simulink model "motor"  (R2020b)
settings: Solver=ode45  StartTime=0.0  StopTime=33  RelTol=1e-3  EnableMultiTasking=on
PreLoadFcn:
  | MotorParam
InitFcn:
  | MotorParam
values from neighbouring files (symbols this model uses):
  B = (Km*INL)/w    (= 5.6014073536e-07)    [MotorParam.m]
  J = Rotor_inertia    (= 5.33664e-07)    [MotorParam.m]
  Kb = (Speed_constant)/(.10472)    (= 0.0279218545472)    [MotorParam.m]
  Km = Torque_constant*1E-3    (= 0.028)    [MotorParam.m]
  L = Terminal_inductance*1E-3    (= 0.000535)    [MotorParam.m]
  R = Terminal_resistance    (= 8.75)    [MotorParam.m]
libraries: simulink x1
settings Model: Creator=Leo  LastModifiedBy=Jeff
settings DataIOCC: LimitDataPoints=on  SaveFormat=Array  SignalLoggingSaveFormat=ModelDataLogs  ReturnWorkspaceOutputs=off
settings OptimizationCC: ExpressionDepthLimit=2147483647  InitFltsAndDblsToZero=on  LifeSpan=inf
settings DebuggingCC: UnderspecifiedInitializationDetection=Classic  MergeDetectMultiDrivingBlocksExec=none  SolverPrmCheckMsg=warning  FcnCallInpInsideContextMsg=warning  StateNameClashWarn=warning  SFUnexpectedBacktrackingDiag=warning  SFNoUnconditionalDefaultTransitionDiag=warning  SFExecutionAtInitializationDiag=none  ArithmeticOperatorsInVariantConditions=warning
settings HardwareCC: ProdBitPerPointer=32  ProdBitPerSizeT=32  ProdBitPerPtrDiffT=32  ProdLargestAtomicFloat=None  ProdIntDivRoundTo=Undefined  ProdEndianess=Unspecified  ProdWordSize=32  ProdHWDeviceType=32-bit Generic
settings ModelReferenceCC: PropagateSignalLabelsOutOfModel=off
settings SFSimCC: SimUseLocalCustomCode=off  CustomCodeUndefinedFunction=UseInterfaceOnly
settings RTWCC: RTWUseLocalCustomCode=off
settings CodeAppCC: StateflowObjectComments=on
settings GRTTargetCC: TargetLangStandard=C89/C90 (ANSI)  CombineOutputUpdateFcns=off  GRTInterface=on
settings ConfigComp: CovMetricSettings=dw  CovSaveCumulativeToWorkspaceVar=on  CovSaveSingleToWorkspaceVar=on  CovExternalEMLEnable=off  CovSFcnEnable=off

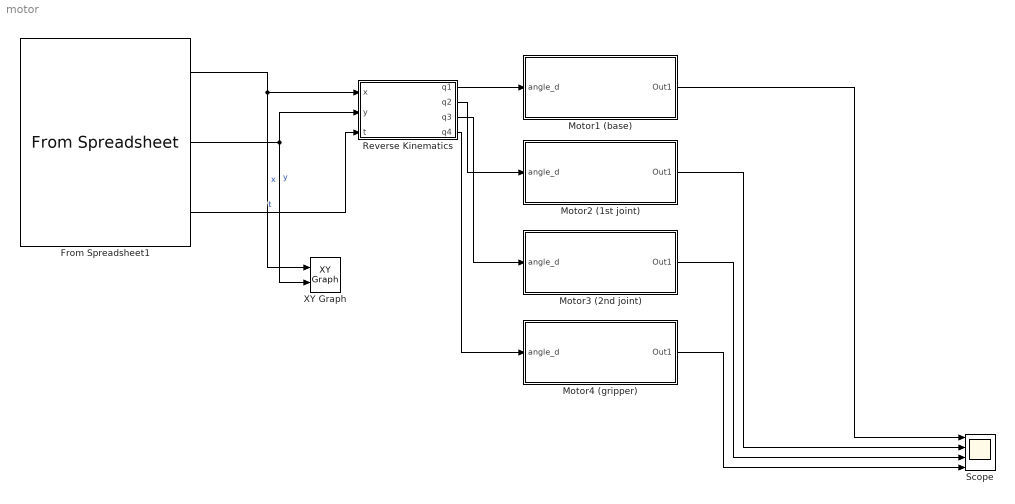
== system motor ==
  From Spreadsheet1 : FromSpreadsheet  FileName=Motor_pos.xlsx
  Motor1 (base) : Subsystem
  Motor2 (1st joint) : Subsystem
  Motor3 (2nd joint) : Subsystem
  Motor4 (gripper) : Subsystem
  Reverse Kinematics : MATLAB Function  TreatAsAtomicUnit=on
  Scope : Scope  NumInputPorts=4
  XY Graph : simulink/Sinks/XY Graph  xmin=-15  xmax=15  ymin=-5  ymax=50  st=0.001
  wires:
  From Spreadsheet1/1 -> XY Graph/1, Reverse Kinematics/1(x)  "x"
  Motor1 (base)/1(Out1) -> Scope/1
  From Spreadsheet1/2 -> XY Graph/2, Reverse Kinematics/2(y)  "y"
  Reverse Kinematics/1(q1) -> Motor1 (base)/1(angle_d)
  Reverse Kinematics/2(q2) -> Motor2 (1st joint)/1(angle_d)
  Reverse Kinematics/3(q3) -> Motor3 (2nd joint)/1(angle_d)
  Motor2 (1st joint)/1(Out1) -> Scope/2
  Motor3 (2nd joint)/1(Out1) -> Scope/3
  Reverse Kinematics/4(q4) -> Motor4 (gripper)/1(angle_d)
  Motor4 (gripper)/1(Out1) -> Scope/4
  From Spreadsheet1/3 -> Reverse Kinematics/3(t)  "t"

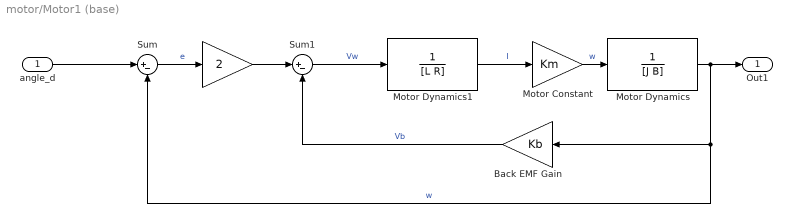
== system motor/Motor1 (base) ==
  angle_d : Inport
  " " : Gain  Gain=2
  Back EMF Gain : Gain  Gain=Kb
  Motor Constant : Gain  Gain=Km
  Motor Dynamics : TransferFcn  Denominator=[J B]
  Motor Dynamics1 : TransferFcn  Denominator=[L R]
  Sum : Sum  Inputs=|+-
  Sum1 : Sum  Inputs=|+-
  Out1 : Outport
  wires:
  angle_d/1 -> Sum/1
  Sum/1 -> " "/1  "e"
  Motor Constant/1 -> Motor Dynamics/1  "w"
  " "/1 -> Sum1/1
  Back EMF Gain/1 -> Sum1/2  "Vb"
  Motor Dynamics1/1 -> Motor Constant/1  "I"
  Sum1/1 -> Motor Dynamics1/1  "Vw"
  Motor Dynamics/1 -> Back EMF Gain/1, Sum/2, Out1/1  "w"

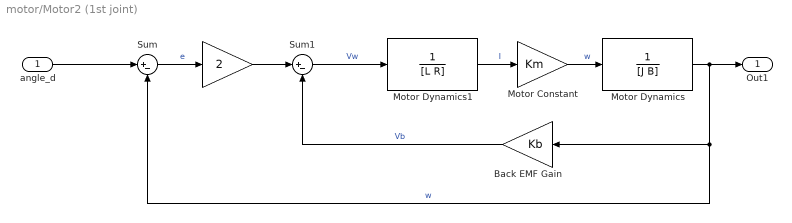
== system motor/Motor2 (1st joint) ==
  angle_d : Inport
  " " : Gain  Gain=2
  Back EMF Gain : Gain  Gain=Kb
  Motor Constant : Gain  Gain=Km
  Motor Dynamics : TransferFcn  Denominator=[J B]
  Motor Dynamics1 : TransferFcn  Denominator=[L R]
  Sum : Sum  Inputs=|+-
  Sum1 : Sum  Inputs=|+-
  Out1 : Outport
  wires:
  Back EMF Gain/1 -> Sum1/2  "Vb"
  Sum/1 -> " "/1  "e"
  Motor Constant/1 -> Motor Dynamics/1  "w"
  " "/1 -> Sum1/1
  Motor Dynamics1/1 -> Motor Constant/1  "I"
  angle_d/1 -> Sum/1
  Sum1/1 -> Motor Dynamics1/1  "Vw"
  Motor Dynamics/1 -> Back EMF Gain/1, Sum/2, Out1/1  "w"

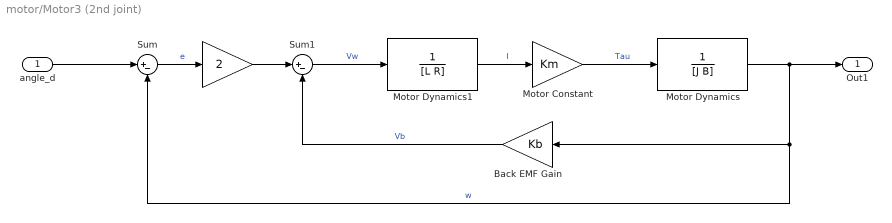
== system motor/Motor3 (2nd joint) ==
  angle_d : Inport
  " " : Gain  Gain=2
  Back EMF Gain : Gain  Gain=Kb
  Motor Constant : Gain  Gain=Km
  Motor Dynamics : TransferFcn  Denominator=[J B]
  Motor Dynamics1 : TransferFcn  Denominator=[L R]
  Sum : Sum  Inputs=|+-
  Sum1 : Sum  Inputs=|+-
  Out1 : Outport
  wires:
  angle_d/1 -> Sum/1
  Sum/1 -> " "/1  "e"
  Motor Dynamics/1 -> Out1/1, Sum/2, Back EMF Gain/1  "w"
  Motor Constant/1 -> Motor Dynamics/1  "Tau"
  " "/1 -> Sum1/1
  Back EMF Gain/1 -> Sum1/2  "Vb"
  Motor Dynamics1/1 -> Motor Constant/1  "I"
  Sum1/1 -> Motor Dynamics1/1  "Vw"

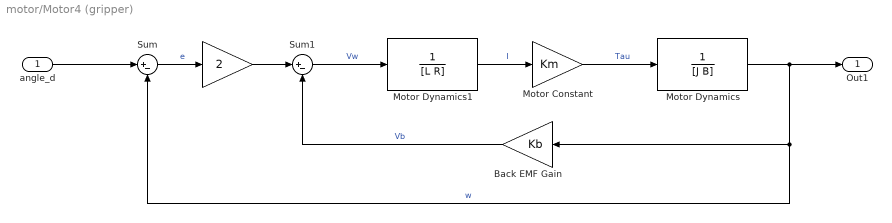
== system motor/Motor4 (gripper) ==
  angle_d : Inport
  " " : Gain  Gain=2
  Back EMF Gain : Gain  Gain=Kb
  Motor Constant : Gain  Gain=Km
  Motor Dynamics : TransferFcn  Denominator=[J B]
  Motor Dynamics1 : TransferFcn  Denominator=[L R]
  Sum : Sum  Inputs=|+-
  Sum1 : Sum  Inputs=|+-
  Out1 : Outport
  wires:
  angle_d/1 -> Sum/1
  Sum/1 -> " "/1  "e"
  Motor Dynamics/1 -> Out1/1, Sum/2, Back EMF Gain/1  "w"
  Motor Constant/1 -> Motor Dynamics/1  "Tau"
  " "/1 -> Sum1/1
  Back EMF Gain/1 -> Sum1/2  "Vb"
  Motor Dynamics1/1 -> Motor Constant/1  "I"
  Sum1/1 -> Motor Dynamics1/1  "Vw"

== matlab function motor/Reverse Kinematics ==
  data: x input; y input; t input; q1 output; q2 output; q3 output; q4 output
    function [q1, q2, q3, q4]= fcn(x,y,t)
    a1 = 20;
    a2 = 30;
    
    q2 = acosd((x^2+y^2-a1^2-a2^2)/(2*a1*a2));
    q1 = atand(y/x)-atand(a2*sind(q2)/(a1+a2*cosd(q2)));
    q4 = 0;
    if q1<0 
        q1 = 180+q1;
    end
    q3 = 180-q1-q2;
    if q3<0
        q3 = 90;
    end
    
    if x==-10 && y==40 && t>=5 && t<=7
        % close gripper
        q4 = 180;
    end
    if x==-10 && y==30 && t>=9 && t<=11
        % open gripper
        q4 = 0;
    end
    
    if x==0 && y==40 && t>=15 && t<=17
        % close gripper
        q4 = 180;
    end
    if x==0 && y==30 && t>=19 && t<=21
        % open gripper
        q4 = 0;
    end
    
    if x==10 && y==40 && t>=25 && t<=27
        % close gripper
        q4 = 180;
    end
    if x==10 && y==30 && t>=29 && t<=31
        % open gripper
        q4 = 0;
    end
